simulink model "V1_model"  (R2024b)
settings: Solver=FixedStepAuto  StartTime=0.0  StopTime=5  FixedStep=0.01  RelTol=1e-3
settings Model: Creator=jz74  LastModifiedBy=shilianshen

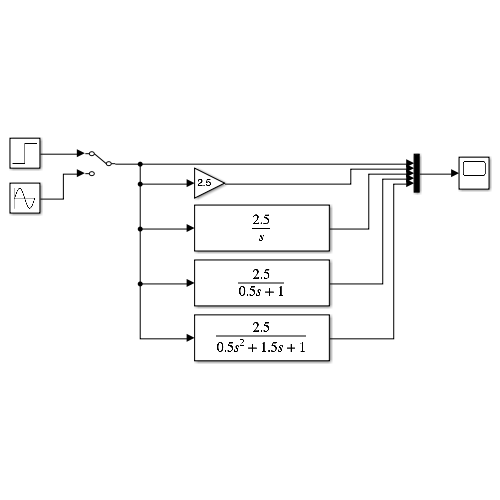
[thumbnail: Simulink's stored preview of the top-level diagram]
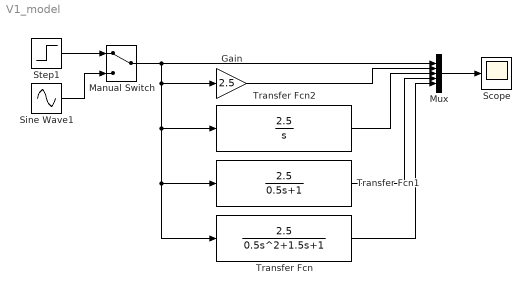
== system V1_model ==
  Gain : Gain  Gain=2.5
  Manual Switch : ManualSwitch
  Mux : Mux  Inputs=5
  Scope : Scope
  Sine Wave1 : Sin  Frequency=5  SampleTime=0
  Step1 : Step  SampleTime=0
  Transfer Fcn : TransferFcn  Numerator=[2.5]  Denominator=[0.5 1.5 1]
  Transfer Fcn1 : TransferFcn  Numerator=[2.5]  Denominator=[0.5 1]
  Transfer Fcn2 : TransferFcn  Numerator=[2.5]  Denominator=[1 0]
  wires:
  Gain/1 -> Mux/2
  Transfer Fcn2/1 -> Mux/3
  Transfer Fcn1/1 -> Mux/4
  Transfer Fcn/1 -> Mux/5
  Mux/1 -> Scope/1
  Manual Switch/1 -> Mux/1, Gain/1, Transfer Fcn/1, Transfer Fcn1/1, Transfer Fcn2/1
  Step1/1 -> Manual Switch/1
  Sine Wave1/1 -> Manual Switch/2
